simulink model "zvt_boost"  (Simulink 6.1)
settings: Solver=ode23tb  StartTime=0.0  StopTime=5e-4  MaxStep=1e-7  RelTol=1e-4  AbsTol=1e-4
libraries: powerlib x10
settings Model: Creator=dkennedy  LastModifiedBy=ThinkPad  ExtModeTrigMode=oneshot  ExtModeArmWhenConnect=off  ExtModeAutoUpdateStatusClock=off
settings DataIOCC: LimitDataPoints=off  SignalLoggingName=sigsOut
settings OptimizationCC: BlockReduction=off  BooleanDataType=off
settings HardwareCC: TargetUnknown=on

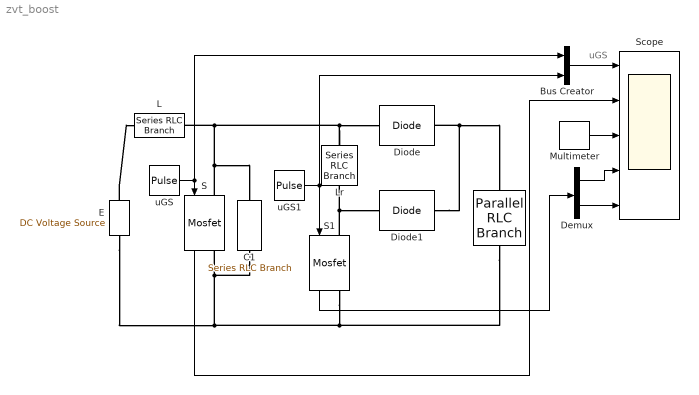
== system zvt_boost ==
  note: uGS
  " " : powerlib/Elements/Parallel RLC Branch  Orientation=down  PhysicalDomain=powersysdomain  SubClassName=unknown  LeftPortType=p1  RightPortType=p1  LConnTagsString=a  RConnTagsString=__new0  Resistance=10  Inductance=inf  Capacitance=1e-5  Measurements=Branch voltage
  Bus Creator : BusCreator  DialogController=Simulink.DDGSource_Bus  Inputs=2
  C1 : powerlib/Elements/Series RLC Branch  Orientation=down  PhysicalDomain=powersysdomain  SubClassName=unknown  LeftPortType=p1  RightPortType=p1  LConnTagsString=__new0  RConnTagsString=__new0  Resistance=0  Inductance=0  Capacitance=5e-8  Measurements=Branch voltage
  Demux : Demux  Outputs=2
  Diode : powerlib/Power Electronics/Diode  Ron=0.001  Lon=0  Vf=0.8  IC=0  Rs=500  Cs=0  Measurements=off
  Diode1 : powerlib/Power Electronics/Diode  Ron=0.001  Lon=0  Vf=0.8  IC=0  Rs=1000  Cs=0  Measurements=off
  E : powerlib/Electrical Sources/DC Voltage Source  Description=source block  Orientation=up  Amplitude=50  Measurements=None
      settings: AttributesFormatString=\n
  L : powerlib/Elements/Series RLC Branch  PhysicalDomain=powersysdomain  SubClassName=unknown  LeftPortType=p1  RightPortType=p1  LConnTagsString=__new0  RConnTagsString=__new0  Resistance=0  Inductance=1e-4  Capacitance=inf  Measurements=Branch current
  Lr : powerlib/Elements/Series RLC Branch  Orientation=down  PhysicalDomain=powersysdomain  SubClassName=unknown  LeftPortType=p1  RightPortType=p1  LConnTagsString=__new0  RConnTagsString=__new0  Resistance=0  Inductance=2e-6  Capacitance=inf  Measurements=Branch current
  Multimeter : powerlib/Measurements/Multimeter  PhasorSimulation=off  OutputType=Complex  sel=[4 3]  L=4  Gain=[1 1]  yselected={'Ib: Lr','Ib: L'};  PSBOutputType=1  PSBequivalent=0  AxesSetting=[0,0.1,-100,100]  Display=0  SavedBlockNames=-11
  S : powerlib/Power Electronics/Mosfet  Orientation=down  Ron=0.01  Lon=1e-9  Rd=.1  IC=0  Rs=100  Cs=1e-8  Measurements=on
  S1 : powerlib/Power Electronics/Mosfet  Orientation=down  Ron=0.01  Lon=1e-8  Rd=.1  IC=0  Rs=10  Cs=1e-9  Measurements=on
  Scope : Scope  NumInputPorts=5
      settings: TimeRange=5e-005  YMin=-1~-50~-10~-10~-50  YMax=2~150~30~30~150  SaveName=var  MaxDataPoints=50000
  uGS : DiscretePulseGenerator  PulseType=Time based  Period=20e-6  PulseWidth=30
  uGS1 : DiscretePulseGenerator  PulseType=Time based  Period=20e-6  PulseWidth=5  PhaseDelay=19e-6
  wires:
  uGS/1 -> S/1, Bus Creator/1
  S/1 -> Scope/2
  Multimeter/1 -> Scope/3
  uGS1/1 -> S1/1, Bus Creator/2
  Bus Creator/1 -> Scope/1
  Demux/1 -> Scope/4
  Demux/2 -> Scope/5
  S1/1 -> Demux/1
  connections:
  S1/RConn1 -- E/LConn1 -- S/RConn1 -- C1/RConn1 -- " "/RConn1
  E/RConn1 -- L/LConn1
  Lr/LConn1 -- S/LConn1 -- C1/LConn1 -- L/RConn1 -- Diode/LConn1
  S1/LConn1 -- Lr/RConn1 -- Diode1/LConn1
  Diode1/RConn1 -- Diode/RConn1 -- " "/LConn1
